simulink model "model"  (R2020a)
settings: Solver=VariableStepAuto  StartTime=0.0  StopTime=10.0  RelTol=1e-3
undefined symbols (not defined in the file): C, R
settings Model: Creator=PRATIKSHA  LastModifiedBy=PRATIKSHA

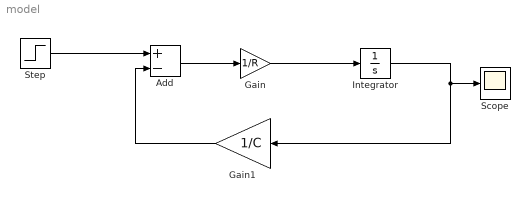
== system model ==
  Add : Sum  Inputs=+-
  Gain : Gain  Gain=1/R
  Gain1 : Gain  Gain=1/C
  Integrator : Integrator  InitialCondition=8
  Scope : Scope
  Step : Step  SampleTime=0
  wires:
  Gain/1 -> Integrator/1
  Gain1/1 -> Add/2
  Add/1 -> Gain/1
  Step/1 -> Add/1
  Integrator/1 -> Gain1/1, Scope/1
